simulink model "Assignment2"  (R2016a)
settings: Solver=VariableStepAuto  StartTime=0.0  StopTime=10.0  RelTol=1e-3
libraries: hdlsllib x1
settings Model: Creator=duyvu  LastModifiedBy=duyvu

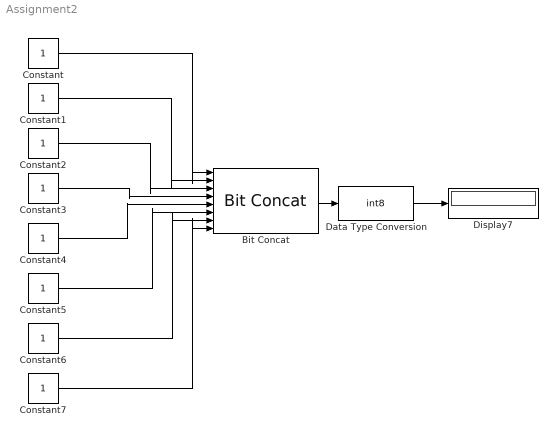
== system Assignment2 ==
  Bit Concat : hdlsllib/HDL Operations/Bit Concat  numInputs=8
  Constant{,1..7} (8 alike) : Constant  OutDataTypeStr=boolean
  Data Type Conversion : DataTypeConversion  OutDataTypeStr=int8  ConvertRealWorld=Stored Integer (SI)
  Display7 : Display
      settings: Format=decimal (Stored Integer)
  wires:
  Bit Concat/1 -> Data Type Conversion/1
  Constant/1 -> Bit Concat/1
  Constant1/1 -> Bit Concat/2
  Constant2/1 -> Bit Concat/3
  Constant3/1 -> Bit Concat/4
  Constant4/1 -> Bit Concat/5
  Constant5/1 -> Bit Concat/6
  Constant6/1 -> Bit Concat/7
  Constant7/1 -> Bit Concat/8
  Data Type Conversion/1 -> Display7/1
